simulink model "PID_control"  (R2024b)
settings: Solver=VariableStepAuto  StartTime=0.0  StopTime=7000  RelTol=1e-3
model workspace (MAT data in the model file):
  Cd = 180
  Csh = 30
  K = 3.1616
  Tauf = 5
  Tf = 8
  Tfuel = 8
  Tw = 6
  k = 3.1616
undefined symbols (not defined in the file): CV_FINAL_VALUE, CV_INIT_VALUE, SIG_FINAL_VALUE, SIG_INIT_VALUE, STEP_TIME
libraries: slpidlib x2
settings Model: Creator=jakub
settings SolverCC: ZeroCrossAlgorithm=Adaptive
settings DebuggingCC: IgnoredZcDiagnostic=none
settings RTWCC: GPUComputeCapability=3.5

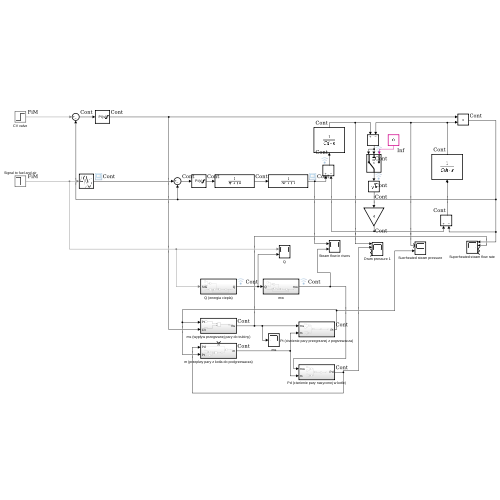
[thumbnail: Simulink's stored preview of the top-level diagram]
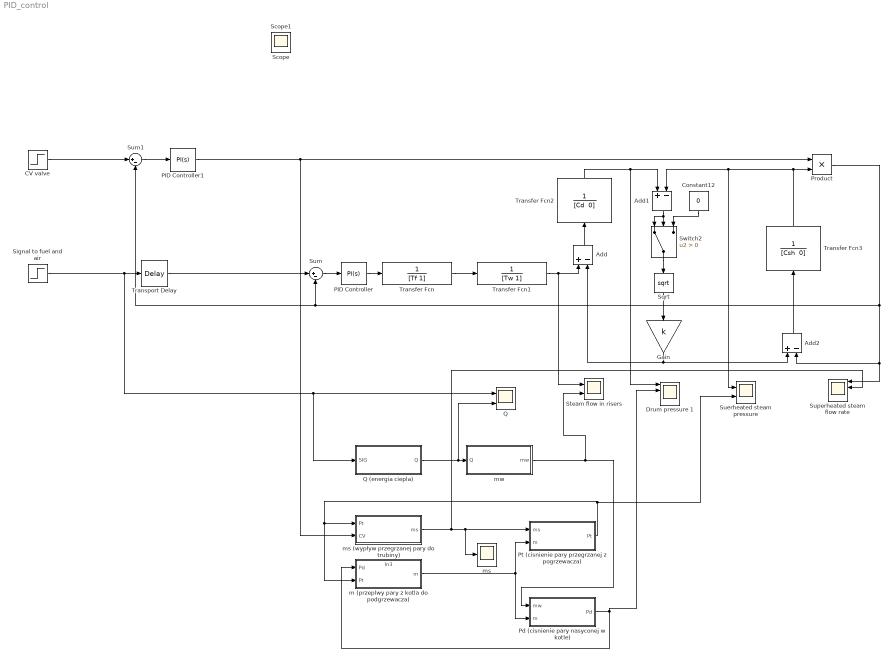
== system PID_control ==
  " mw " : Subsystem
  Add : Sum  Inputs=+-
  Add1 : Sum  Inputs=+-
  Add2 : Sum  Inputs=+-
  CV valve : Step  Time=STEP_TIME  Before=CV_INIT_VALUE  After=CV_FINAL_VALUE  SampleTime=0
  Constant12 : Constant  Value=0
  Drum pressure 1 : Scope  NumInputPorts=4
  Gain : Gain  Gain=k
  PID Controller : slpidlib/PID Controller  Controller=PI  Form=Parallel  TimeDomain=Continuous-time  UseExternalTs=off  SampleTime=-1  IntegratorMethod=Forward Euler  FilterMethod=Forward Euler  ControllerParametersSource=internal  P=3.6  I=0.144  UseKiTs=off  D=400  UseExternalDerivativeSource=off  N=1  UseFilter=on  TunerSelectOption=Transfer Function Based (PID Tuner App)  InitialConditionSource=internal  InitialConditionForIntegrator=0  InitialConditionForFilter=0  DifferentiatorICPrevScaledInput=0  ExternalReset=none  TrackingMode=off  Kt=1  LimitOutput=on  SatLimitsSource=internal  UpperSaturationLimit=1  LowerSaturationLimit=0  LinearizeAsGain=off  AntiWindupMode=clamping  Kb=1  LimitIntegrator=off  UpperIntegratorSaturationLimit=inf  LowerIntegratorSaturationLimit=-inf  POutMin=[]  POutMax=[]  IOutMin=[]  IOutMax=[]  DOutMin=[]  DOutMax=[]  NOutMin=[]  NOutMax=[]  SumOutMin=[]  SumOutMax=[]  SaturationOutMin=[]  SaturationOutMax=[]  PParamMin=[]  PParamMax=[]  IParamMin=[]  IParamMax=[]  DParamMin=[]  DParamMax=[]  NParamMin=[]  NParamMax=[]  KbParamMin=[]  KbParamMax=[]  KtParamMin=[]  KtParamMax=[]  KbOutMin=[]  KbOutMax=[]  KtOutMin=[]  KtOutMax=[]  IntegratorOutMin=[]  IntegratorOutMax=[]  FilterOutMin=[]  FilterOutMax=[]  SumI1OutMin=[]  SumI1OutMax=[]  SumI2OutMin=[]  SumI2OutMax=[]  SumI3OutMin=[]  SumI3OutMax=[]  SumI4OutMin=[]  SumI4OutMax=[]  SumDOutMin=[]  SumDOutMax=[]  DifferentiatorOutMin=[]  DifferentiatorOutMax=[]  FilterDiffOutCoefMin=[]  FilterDiffOutCoefMax=[]  ReciprocalOutMin=[]  ReciprocalOutMax=[]  SumDenOutMin=[]  SumDenOutMax=[]  SumNumOutMin=[]  SumNumOutMax=[]  DivideOutMin=[]  DivideOutMax=[]  UdiffTsProdOutMin=[]  UdiffTsProdOutMax=[]  NTsProdOutMin=[]  NTsProdOutMax=[]  UintegralTsProdOutMin=[]  UintegralTsProdOutMax=[]  UngainTsProdOutMin=[]  UngainTsProdOutMax=[]  ClampingZeroOutDataTypeStr=Inherit: Inherit via back propagation  ClampingZeroOutMin=[]  ClampingZeroOutMax=[]  FilterDenConstantOutDataTypeStr=Inherit: Inherit via back propagation  FilterDenConstantOutMin=[]  FilterDenConstantOutMax=[]  PCopyOutDataTypeStr=Inherit: Inherit via back propagation  PCopyOutMin=[]  PCopyOutMax=[]  NCopyOutDataTypeStr=Inherit: Inherit via back propagation  NCopyOutMin=[]  NCopyOutMax=[]  IntegratorContinuousStateAttributes=''  IntegratorStateMustResolveToSignalObject=off  IntegratorRTWStateStorageClass=Auto  FilterContinuousStateAttributes=''  FilterStateMustResolveToSignalObject=off  FilterRTWStateStorageClass=Auto  ParallelPVariant=InternalParameters  IdealPVariant=Disabled  IVariant=InternalParameters  DVariant=Disabled  IntegratorVariant=Continuous  SatVariant=Enabled  AWVariant=ContClampingParallel  PCopyVariant=Disabled  TRVariant=Disabled  FdbkBlocksVariant=Forward  IdealPFdbkVariant=Disabled  SatFdbkVariant=Disabled  DerivativeFilterVariant=Disabled  NVariant=Disabled  NCopyVariant=Disabled_SignalSpec  FilterICVariant=Disabled  IntegratorICVariant=InternalICs  ExternalResetVariant=Disabled  TRSumVariant=Passthrough  SumFdbkVariant=Disabled  SumVariant=Sum_PI  TsampFilterVariant=InternalTs  TsampNgainVariant=Passthrough  TsampIntegralVariant=Disabled_SignalSpec  ExternalSaturationOutDataTypeStr=Inherit: Same as second input  DerivativeSourceVariant=Disabled  PreIntVariant=InternalPreInt
  PID Controller1 : slpidlib/PID Controller  Controller=PI  Form=Parallel  TimeDomain=Continuous-time  UseExternalTs=off  SampleTime=-1  IntegratorMethod=Forward Euler  FilterMethod=Forward Euler  ControllerParametersSource=internal  P=1  I=0.1  UseKiTs=off  D=400  UseExternalDerivativeSource=off  N=100  UseFilter=on  TunerSelectOption=Transfer Function Based (PID Tuner App)  InitialConditionSource=internal  InitialConditionForIntegrator=0  InitialConditionForFilter=0  DifferentiatorICPrevScaledInput=0  ExternalReset=none  TrackingMode=off  Kt=1  LimitOutput=on  SatLimitsSource=internal  UpperSaturationLimit=1  LowerSaturationLimit=0  LinearizeAsGain=on  AntiWindupMode=clamping  Kb=1  LimitIntegrator=off  UpperIntegratorSaturationLimit=inf  LowerIntegratorSaturationLimit=-inf  POutMin=[]  POutMax=[]  IOutMin=[]  IOutMax=[]  DOutMin=[]  DOutMax=[]  NOutMin=[]  NOutMax=[]  SumOutMin=[]  SumOutMax=[]  SaturationOutMin=[]  SaturationOutMax=[]  PParamMin=[]  PParamMax=[]  IParamMin=[]  IParamMax=[]  DParamMin=[]  DParamMax=[]  NParamMin=[]  NParamMax=[]  KbParamMin=[]  KbParamMax=[]  KtParamMin=[]  KtParamMax=[]  KbOutMin=[]  KbOutMax=[]  KtOutMin=[]  KtOutMax=[]  IntegratorOutMin=[]  IntegratorOutMax=[]  FilterOutMin=[]  FilterOutMax=[]  SumI1OutMin=[]  SumI1OutMax=[]  SumI2OutMin=[]  SumI2OutMax=[]  SumI3OutMin=[]  SumI3OutMax=[]  SumI4OutMin=[]  SumI4OutMax=[]  SumDOutMin=[]  SumDOutMax=[]  DifferentiatorOutMin=[]  DifferentiatorOutMax=[]  FilterDiffOutCoefMin=[]  FilterDiffOutCoefMax=[]  ReciprocalOutMin=[]  ReciprocalOutMax=[]  SumDenOutMin=[]  SumDenOutMax=[]  SumNumOutMin=[]  SumNumOutMax=[]  DivideOutMin=[]  DivideOutMax=[]  UdiffTsProdOutMin=[]  UdiffTsProdOutMax=[]  NTsProdOutMin=[]  NTsProdOutMax=[]  UintegralTsProdOutMin=[]  UintegralTsProdOutMax=[]  UngainTsProdOutMin=[]  UngainTsProdOutMax=[]  ClampingZeroOutDataTypeStr=Inherit: Inherit via back propagation  ClampingZeroOutMin=[]  ClampingZeroOutMax=[]  FilterDenConstantOutDataTypeStr=Inherit: Inherit via back propagation  FilterDenConstantOutMin=[]  FilterDenConstantOutMax=[]  PCopyOutDataTypeStr=Inherit: Inherit via back propagation  PCopyOutMin=[]  PCopyOutMax=[]  NCopyOutDataTypeStr=Inherit: Inherit via back propagation  NCopyOutMin=[]  NCopyOutMax=[]  IntegratorContinuousStateAttributes=''  IntegratorStateMustResolveToSignalObject=off  IntegratorRTWStateStorageClass=Auto  FilterContinuousStateAttributes=''  FilterStateMustResolveToSignalObject=off  FilterRTWStateStorageClass=Auto  ParallelPVariant=InternalParameters  IdealPVariant=Disabled  IVariant=InternalParameters  DVariant=Disabled  IntegratorVariant=Continuous  SatVariant=Enabled  AWVariant=ContClampingParallel  PCopyVariant=Disabled  TRVariant=Disabled  FdbkBlocksVariant=Forward  IdealPFdbkVariant=Disabled  SatFdbkVariant=Disabled  DerivativeFilterVariant=Disabled  NVariant=Disabled  NCopyVariant=Disabled_SignalSpec  FilterICVariant=Disabled  IntegratorICVariant=InternalICs  ExternalResetVariant=Disabled  TRSumVariant=Passthrough  SumFdbkVariant=Disabled  SumVariant=Sum_PI  TsampFilterVariant=InternalTs  TsampNgainVariant=Passthrough  TsampIntegralVariant=Disabled_SignalSpec  ExternalSaturationOutDataTypeStr=Inherit: Same as second input  DerivativeSourceVariant=Disabled  PreIntVariant=InternalPreInt
  Pd (cisnienie pary nasyconej w kotle) : Subsystem
  Product : Product
  Pt (cisnienie pary przegrzanej z pogrzewacza) : Subsystem
  Q : Scope  NumInputPorts=2
  Q (energia ciepla) : Subsystem
  Signal to fuel and air : Step  Time=STEP_TIME  Before=SIG_INIT_VALUE  After=SIG_FINAL_VALUE  SampleTime=0
  Sqrt : Sqrt
  Steam flow in risers : Scope  NumInputPorts=2
  Suerheated steam pressure : Scope  NumInputPorts=2
  Sum : Sum  Inputs=|+-
  Sum1 : Sum  Inputs=|+-
  Superheated steam flow rate : Scope  NumInputPorts=4
  Switch2 : Switch  Criteria=u2 > Threshold  SaturateOnIntegerOverflow=off  InputSameDT=off
  Transfer Fcn : TransferFcn  Denominator=[Tf 1]
  Transfer Fcn1 : TransferFcn  Denominator=[Tw 1]
  Transfer Fcn2 : TransferFcn  Denominator="[Cd  0]"
  Transfer Fcn3 : TransferFcn  Denominator="[Csh  0]"
  Transport Delay : TransportDelay  DelayTime=Tauf
  m (przeplwy pary z kotla do podgrzewacza) : Subsystem
      settings: PortSchema="{\"entries\":[{\"content\":{\"sides\":[{\"content\":{\"connectorIds\":[\"In1\",\"In2\"]},\"type\":\"ConnectorPlacement.EquallySpacedRectSide\",\"uuid\":\"cfa7c649-b017-4d3e-928d-e86863ec027a\"},{\"content\":{\"connectorIds\":[\"Out1\"],\"side\":\"RIGHT\"},\"type\":\"ConnectorPlacement.EquallySpacedRectSide\",\"uuid\":\"fe8bf8f7-b818-41d4-92f6-ee3a6490ff89\"},{\"content\":{\"connectorIds\":[\"In3\"],\"side\":\"TOP\"},\"type\":\"ConnectorPlacement.EquallySpacedRectSide\",\"uuid\":\"62e4c2c3-fda5-4519-817f-132425e1dc36\"}]},\"type\":\"ConnectorPlacement.EquallySpacedConnector\",\"uuid\":\"cd14fa44-292b-40ad-89b9-6a37a56970f2\"}],\"packageUris\":[\"http://schema.mathworks.com/mf0/Connector/R2020b\"],\"version\":\"1.0\"}"
  ms : Scope
  ms (wypływ przegrzanej pary do trubiny) : Subsystem
  Scope : Scope
  Scope1 : Scope
  wires:
  Transfer Fcn3/1 -> Suerheated steam pressure/1, Add1/2, Product/2
  Add2/1 -> Transfer Fcn3/1
  Gain/1 -> Add2/1, Add/2
  Transport Delay/1 -> Sum/1
  Signal to fuel and air/1 -> Transport Delay/1, Q/1, Q (energia ciepla)/1(SIG)
  Transfer Fcn2/1 -> Drum pressure 1/1, Add1/1
  Transfer Fcn1/1 -> Steam flow in risers/1, Add/1
  Add/1 -> Transfer Fcn2/1
  Sqrt/1 -> Gain/1
  Transfer Fcn/1 -> Transfer Fcn1/1
  Q (energia ciepla)/1(Q) -> Q/2, " mw "/1(Q)
  ms (wypływ przegrzanej pary do trubiny)/1(ms) -> Superheated steam flow rate/2, ms/1, Pt (cisnienie pary przegrzanej z pogrzewacza)/1(ms)
  Pt (cisnienie pary przegrzanej z pogrzewacza)/1(Pt) -> Suerheated steam pressure/2, ms (wypływ przegrzanej pary do trubiny)/1(Pt), m (przeplwy pary z kotla do podgrzewacza)/2(Pt)
  m (przeplwy pary z kotla do podgrzewacza)/1(m) -> Pd (cisnienie pary nasyconej w kotle)/2(m), Pt (cisnienie pary przegrzanej z pogrzewacza)/2(m)
  " mw "/1(mw) -> Steam flow in risers/2, Pd (cisnienie pary nasyconej w kotle)/1(mw)
  Pd (cisnienie pary nasyconej w kotle)/1(Pd) -> m (przeplwy pary z kotla do podgrzewacza)/1(Pd), Drum pressure 1/2
  Add1/1 -> Switch2/1, Switch2/2
  Switch2/1 -> Sqrt/1
  Constant12/1 -> Switch2/3
  Sum/1 -> PID Controller/1
  Product/1 -> Sum1/2, Sum/2, Superheated steam flow rate/1, Add2/2
  PID Controller1/1 -> Product/1, ms (wypływ przegrzanej pary do trubiny)/2(CV)
  PID Controller/1 -> Transfer Fcn/1
  CV valve/1 -> Sum1/1
  Sum1/1 -> PID Controller1/1

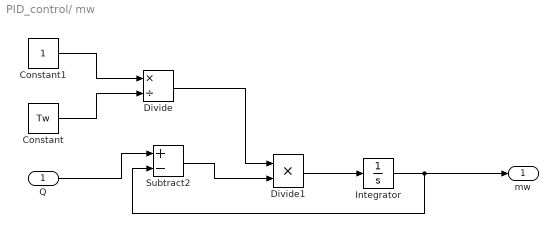
== system PID_control/ mw  ==
  Q : Inport
  Constant : Constant  Value=Tw
  Constant1 : Constant
  Divide : Product  Inputs=*/
  Divide1 : Product  Inputs=**  RndMeth=Zero  SaturateOnIntegerOverflow=on
  Integrator : Integrator
  Subtract2 : Sum  Inputs=+-
  mw : Outport
  wires:
  Divide/1 -> Divide1/1
  Constant1/1 -> Divide/1
  Constant/1 -> Divide/2
  Divide1/1 -> Integrator/1
  Integrator/1 -> Subtract2/2, mw/1
  Q/1 -> Subtract2/1
  Subtract2/1 -> Divide1/2

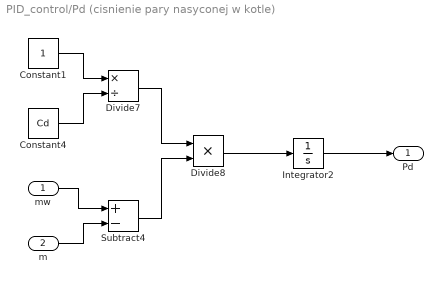
== system PID_control/Pd (cisnienie pary nasyconej w kotle) ==
  mw : Inport
  m : Inport  Port=2
  Constant1 : Constant
  Constant4 : Constant  Value=Cd
  Divide7 : Product  Inputs=*/
  Divide8 : Product  Inputs=**
  Integrator2 : Integrator
  Subtract4 : Sum  Inputs=+-
  Pd : Outport
  wires:
  mw/1 -> Subtract4/1
  m/1 -> Subtract4/2
  Constant4/1 -> Divide7/2
  Constant1/1 -> Divide7/1
  Subtract4/1 -> Divide8/2
  Divide7/1 -> Divide8/1
  Divide8/1 -> Integrator2/1
  Integrator2/1 -> Pd/1

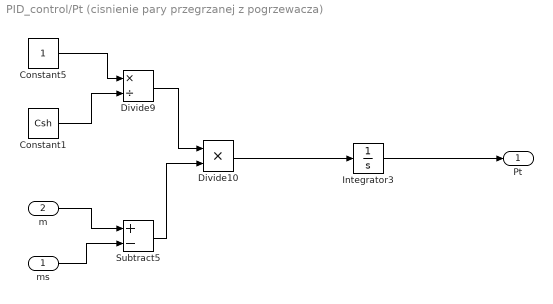
== system PID_control/Pt (cisnienie pary przegrzanej z pogrzewacza) ==
  ms : Inport
  m : Inport  Port=2
  Constant1 : Constant  Value=Csh
  Constant5 : Constant
  Divide10 : Product  Inputs=**
  Divide9 : Product  Inputs=*/
  Integrator3 : Integrator
  Subtract5 : Sum  Inputs=+-
  Pt : Outport
  wires:
  ms/1 -> Subtract5/2
  m/1 -> Subtract5/1
  Constant1/1 -> Divide9/2
  Constant5/1 -> Divide9/1
  Divide9/1 -> Divide10/1
  Subtract5/1 -> Divide10/2
  Divide10/1 -> Integrator3/1
  Integrator3/1 -> Pt/1

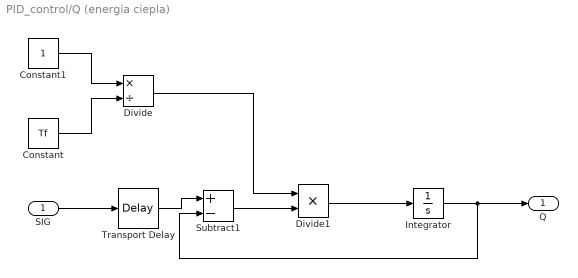
== system PID_control/Q (energia ciepla) ==
  SIG : Inport
  Constant : Constant  Value=Tf
  Constant1 : Constant
  Divide : Product  Inputs=*/
  Divide1 : Product  Inputs=**  RndMeth=Zero  SaturateOnIntegerOverflow=on
  Integrator : Integrator
  Subtract1 : Sum  Inputs=+-
  Transport Delay : TransportDelay  DelayTime=Tauf
  Q : Outport
  wires:
  SIG/1 -> Transport Delay/1
  Transport Delay/1 -> Subtract1/1
  Subtract1/1 -> Divide1/2
  Constant1/1 -> Divide/1
  Constant/1 -> Divide/2
  Divide/1 -> Divide1/1
  Divide1/1 -> Integrator/1
  Integrator/1 -> Subtract1/2, Q/1

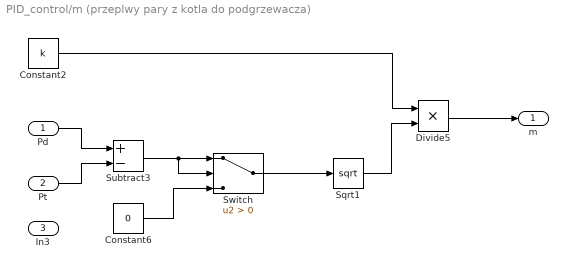
== system PID_control/m (przeplwy pary z kotla do podgrzewacza) ==
  Pd : Inport
  Pt : Inport  Port=2
  In3 : Inport  Port=3
  Constant2 : Constant  Value=k
  Constant6 : Constant  Value=0
  Divide5 : Product  Inputs=**
  Sqrt1 : Sqrt
  Subtract3 : Sum  Inputs=+-
  Switch : Switch  Criteria=u2 > Threshold  SaturateOnIntegerOverflow=off  InputSameDT=off
  m : Outport
  wires:
  Pd/1 -> Subtract3/1
  Pt/1 -> Subtract3/2
  Constant6/1 -> Switch/3
  Subtract3/1 -> Switch/1, Switch/2
  Switch/1 -> Sqrt1/1
  Constant2/1 -> Divide5/1
  Sqrt1/1 -> Divide5/2
  Divide5/1 -> m/1

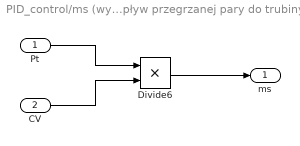
== system PID_control/ms (wypływ przegrzanej pary do trubiny) ==
  Pt : Inport
  CV : Inport  Port=2
  Divide6 : Product  Inputs=**
  ms : Outport
  wires:
  Pt/1 -> Divide6/1
  CV/1 -> Divide6/2
  Divide6/1 -> ms/1
